simulink model "TST_Prp_TrqDesCoord"  (R2016b)
settings: Solver=FixedStepDiscrete  StartTime=0.0  StopTime=simTime  FixedStep=sampleTime  RelTol=1e-3
values from neighbouring files (symbols this model uses):
  testCase = 1    [initTST_Prp_TrqDesCoord_001.m]
libraries: simulink x2
settings Model: Creator=WF305  LastModifiedBy=WF305
settings DebuggingCC: SignalRangeChecking=error

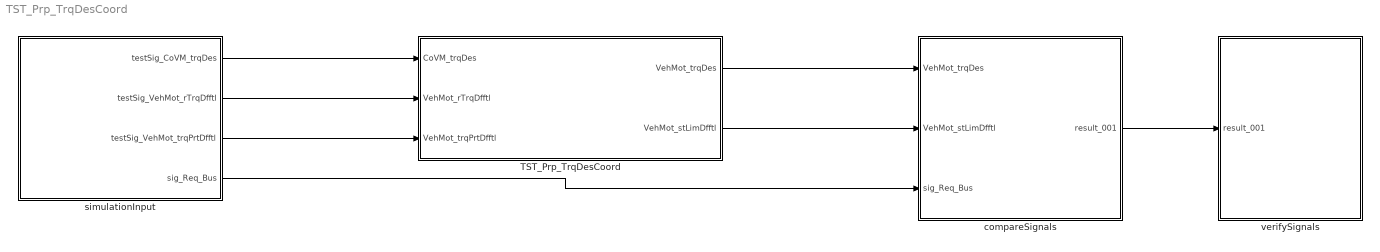
== system TST_Prp_TrqDesCoord ==
  TST_Prp_TrqDesCoord : Subsystem
  compareSignals : Subsystem
  simulationInput : Subsystem
  verifySignals : Subsystem
  wires:
  simulationInput/1(testSig_CoVM_trqDes) -> TST_Prp_TrqDesCoord/1(CoVM_trqDes)
  simulationInput/2(testSig_VehMot_rTrqDfftl) -> TST_Prp_TrqDesCoord/2(VehMot_rTrqDfftl)
  simulationInput/3(testSig_VehMot_trqPrtDfftl) -> TST_Prp_TrqDesCoord/3(VehMot_trqPrtDfftl)
  TST_Prp_TrqDesCoord/1(VehMot_trqDes) -> compareSignals/1(VehMot_trqDes)
  TST_Prp_TrqDesCoord/2(VehMot_stLimDfftl) -> compareSignals/2(VehMot_stLimDfftl)
  simulationInput/4(sig_Req_Bus) -> compareSignals/3(sig_Req_Bus)
  compareSignals/1(result_001) -> verifySignals/1(result_001)

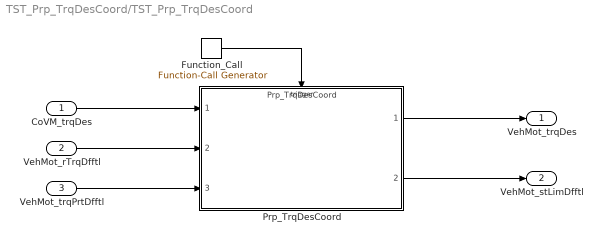
== system TST_Prp_TrqDesCoord/TST_Prp_TrqDesCoord ==
  CoVM_trqDes : Inport
  VehMot_rTrqDfftl : Inport  Port=2
  VehMot_trqPrtDfftl : Inport  Port=3
  Function_Call : simulink/Ports & Subsystems/Function-Call Generator  sample_time=sampleTime  numberOfIterations=1
  Prp_TrqDesCoord : ModelReference  ModelNameDialog=Prp_TrqDesCoord  ModelReferenceVersion=1.3  TriggerPortName=function  TriggerPortTriggerType=function-call  TriggerPortStatesWhenEnabling=held
  VehMot_trqDes : Outport
  VehMot_stLimDfftl : Outport  Port=2
  wires:
  Function_Call/1 -> Prp_TrqDesCoord/Trigger
  CoVM_trqDes/1 -> Prp_TrqDesCoord/1
  VehMot_rTrqDfftl/1 -> Prp_TrqDesCoord/2
  VehMot_trqPrtDfftl/1 -> Prp_TrqDesCoord/3
  Prp_TrqDesCoord/1 -> VehMot_trqDes/1
  Prp_TrqDesCoord/2 -> VehMot_stLimDfftl/1

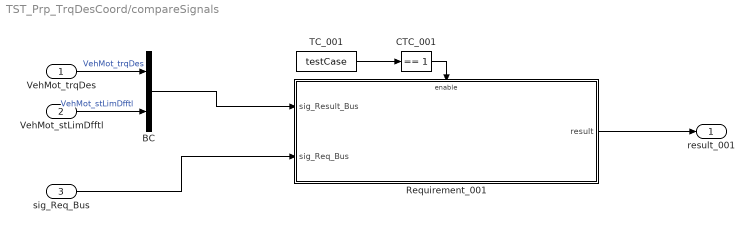
== system TST_Prp_TrqDesCoord/compareSignals ==
  VehMot_trqDes : Inport
  VehMot_stLimDfftl : Inport  Port=2
  sig_Req_Bus : Inport  Port=3
  BC : BusCreator  Inputs=2
  CTC_001 : simulink/Logic and Bit Operations/Compare To Constant  relop===  const=1  OutDataTypeStr=boolean
  Requirement_001 : Subsystem
  TC_001 : Constant  Value=testCase
  result_001 : Outport
  wires:
  VehMot_trqDes/1 -> BC/1  "VehMot_trqDes"
  VehMot_stLimDfftl/1 -> BC/2  "VehMot_stLimDfftl"
  TC_001/1 -> CTC_001/1
  CTC_001/1 -> Requirement_001/Enable
  sig_Req_Bus/1 -> Requirement_001/2(sig_Req_Bus)
  BC/1 -> Requirement_001/1(sig_Result_Bus)
  Requirement_001/1(result) -> result_001/1

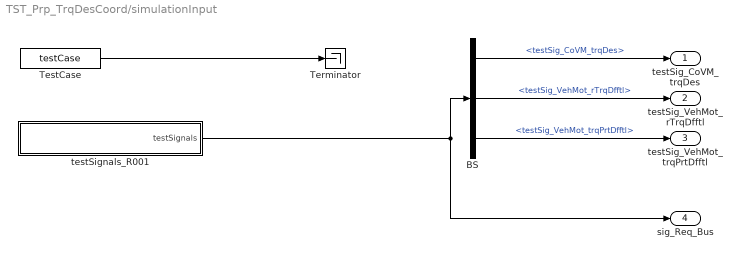
== system TST_Prp_TrqDesCoord/simulationInput ==
  BS : BusSelector  OutputSignals=testSig_CoVM_trqDes,testSig_VehMot_rTrqDfftl,testSig_VehMot_trqPrtDfftl
  Terminator : Terminator
  TestCase : Constant  Value=testCase
  testSignals_R001 : Subsystem
  testSig_CoVM_trqDes : Outport
  testSig_VehMot_rTrqDfftl : Outport  Port=2
  testSig_VehMot_trqPrtDfftl : Outport  Port=3
  sig_Req_Bus : Outport  Port=4
  wires:
  BS/1 -> testSig_CoVM_trqDes/1  "<testSig_CoVM_trqDes>"
  BS/2 -> testSig_VehMot_rTrqDfftl/1  "<testSig_VehMot_rTrqDfftl>"
  BS/3 -> testSig_VehMot_trqPrtDfftl/1  "<testSig_VehMot_trqPrtDfftl>"
  testSignals_R001/1(testSignals) -> BS/1, sig_Req_Bus/1
  TestCase/1 -> Terminator/1

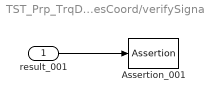
== system TST_Prp_TrqDesCoord/verifySignals ==
  result_001 : Inport
  Assertion_001 : Assertion
  wires:
  result_001/1 -> Assertion_001/1

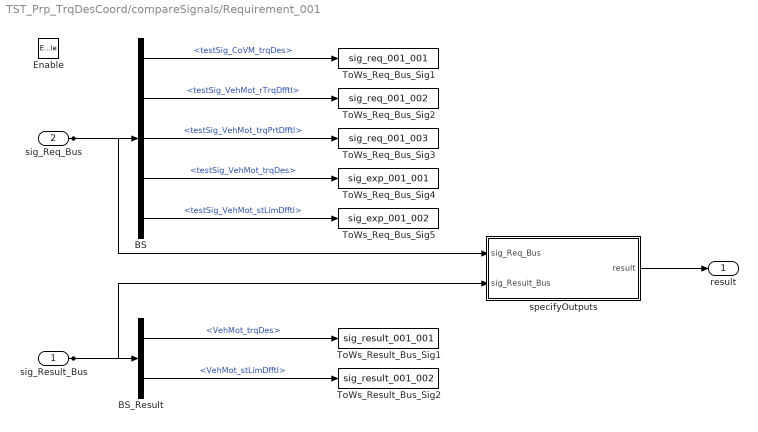
== system TST_Prp_TrqDesCoord/compareSignals/Requirement_001 ==
  sig_Result_Bus : Inport
  sig_Req_Bus : Inport  Port=2
  Enable : EnablePort
  BS : BusSelector  OutputSignals=testSig_CoVM_trqDes,testSig_VehMot_rTrqDfftl,testSig_VehMot_trqPrtDfftl,testSig_VehMot_trqDes,testSig_VehMot_stLimDfftl
  BS_Result : BusSelector  OutputSignals=VehMot_trqDes,VehMot_stLimDfftl
  ToWs_Req_Bus_Sig1 : ToWorkspace  VariableName=sig_req_001_001  SaveFormat=Structure With Time
  ToWs_Req_Bus_Sig2 : ToWorkspace  VariableName=sig_req_001_002  SaveFormat=Structure With Time
  ToWs_Req_Bus_Sig3 : ToWorkspace  VariableName=sig_req_001_003  SaveFormat=Structure With Time
  ToWs_Req_Bus_Sig4 : ToWorkspace  VariableName=sig_exp_001_001  SaveFormat=Structure With Time
  ToWs_Req_Bus_Sig5 : ToWorkspace  VariableName=sig_exp_001_002  SaveFormat=Structure With Time
  ToWs_Result_Bus_Sig1 : ToWorkspace  VariableName=sig_result_001_001  SaveFormat=Structure With Time
  ToWs_Result_Bus_Sig2 : ToWorkspace  VariableName=sig_result_001_002  SaveFormat=Structure With Time
  specifyOutputs : Subsystem
  result : Outport
  wires:
  sig_Req_Bus/1 -> BS/1, specifyOutputs/1(sig_Req_Bus)
  BS/1 -> ToWs_Req_Bus_Sig1/1  "<testSig_CoVM_trqDes>"
  BS/2 -> ToWs_Req_Bus_Sig2/1  "<testSig_VehMot_rTrqDfftl>"
  BS/3 -> ToWs_Req_Bus_Sig3/1  "<testSig_VehMot_trqPrtDfftl>"
  BS/4 -> ToWs_Req_Bus_Sig4/1  "<testSig_VehMot_trqDes>"
  BS/5 -> ToWs_Req_Bus_Sig5/1  "<testSig_VehMot_stLimDfftl>"
  sig_Result_Bus/1 -> BS_Result/1, specifyOutputs/2(sig_Result_Bus)
  BS_Result/1 -> ToWs_Result_Bus_Sig1/1  "<VehMot_trqDes>"
  BS_Result/2 -> ToWs_Result_Bus_Sig2/1  "<VehMot_stLimDfftl>"
  specifyOutputs/1(result) -> result/1

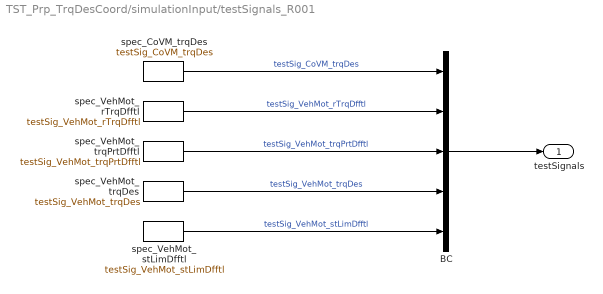
== system TST_Prp_TrqDesCoord/simulationInput/testSignals_R001 ==
  BC : BusCreator  Inputs=5
  spec_CoVM_trqDes : FromWorkspace  VariableName=testSig_CoVM_trqDes  Interpolate=off  OutputAfterFinalValue=Holding final value
  spec_VehMot_rTrqDfftl : FromWorkspace  VariableName=testSig_VehMot_rTrqDfftl  Interpolate=off  OutputAfterFinalValue=Holding final value
  spec_VehMot_stLimDfftl : FromWorkspace  VariableName=testSig_VehMot_stLimDfftl  Interpolate=off  OutputAfterFinalValue=Holding final value
  spec_VehMot_trqDes : FromWorkspace  VariableName=testSig_VehMot_trqDes  Interpolate=off  OutputAfterFinalValue=Holding final value
  spec_VehMot_trqPrtDfftl : FromWorkspace  VariableName=testSig_VehMot_trqPrtDfftl  Interpolate=off  OutputAfterFinalValue=Holding final value
  testSignals : Outport
  wires:
  BC/1 -> testSignals/1
  spec_CoVM_trqDes/1 -> BC/1  "testSig_CoVM_trqDes"
  spec_VehMot_rTrqDfftl/1 -> BC/2  "testSig_VehMot_rTrqDfftl"
  spec_VehMot_trqPrtDfftl/1 -> BC/3  "testSig_VehMot_trqPrtDfftl"
  spec_VehMot_trqDes/1 -> BC/4  "testSig_VehMot_trqDes"
  spec_VehMot_stLimDfftl/1 -> BC/5  "testSig_VehMot_stLimDfftl"

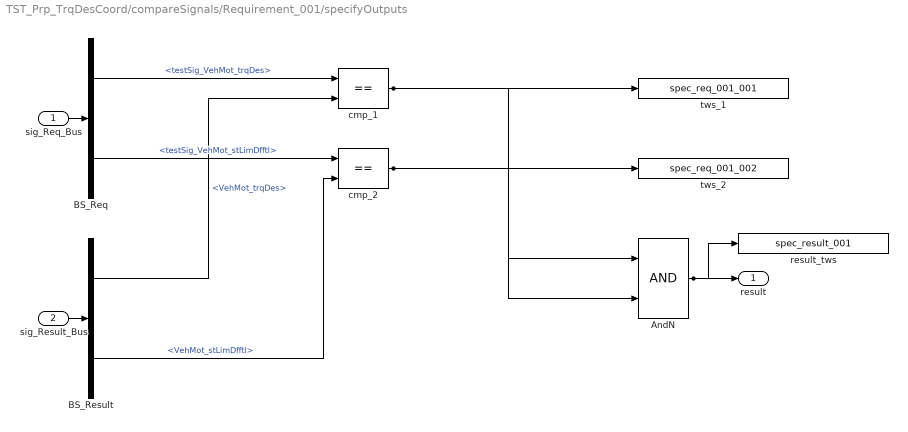
== system TST_Prp_TrqDesCoord/compareSignals/Requirement_001/specifyOutputs ==
  sig_Req_Bus : Inport
  sig_Result_Bus : Inport  Port=2
  AndN : Logic
  BS_Req : BusSelector  OutputSignals=testSig_VehMot_trqDes,testSig_VehMot_stLimDfftl
  BS_Result : BusSelector  OutputSignals=VehMot_trqDes,VehMot_stLimDfftl
  cmp_1 : RelationalOperator  Operator===  RndMeth=Nearest  InputSameDT=on
  cmp_2 : RelationalOperator  Operator===  RndMeth=Nearest  InputSameDT=on
  result_tws : ToWorkspace  VariableName=spec_result_001
  tws_1 : ToWorkspace  VariableName=spec_req_001_001
  tws_2 : ToWorkspace  VariableName=spec_req_001_002
  result : Outport
  wires:
  sig_Req_Bus/1 -> BS_Req/1
  sig_Result_Bus/1 -> BS_Result/1
  AndN/1 -> result/1, result_tws/1
  BS_Req/1 -> cmp_1/1  "<testSig_VehMot_trqDes>"
  BS_Result/1 -> cmp_1/2  "<VehMot_trqDes>"
  cmp_1/1 -> tws_1/1, AndN/1
  BS_Req/2 -> cmp_2/1  "<testSig_VehMot_stLimDfftl>"
  BS_Result/2 -> cmp_2/2  "<VehMot_stLimDfftl>"
  cmp_2/1 -> tws_2/1, AndN/2
